simulink model "scheme1"  (R2024a)
settings: Solver=VariableStepAuto  StartTime=0.0  StopTime=inf  RelTol=1e-9
undefined symbols (not defined in the file): J, ke, km, R
libraries: instrumentseriallib x2
settings Model: Creator=alexivanov  LastModifiedBy=alexivanov

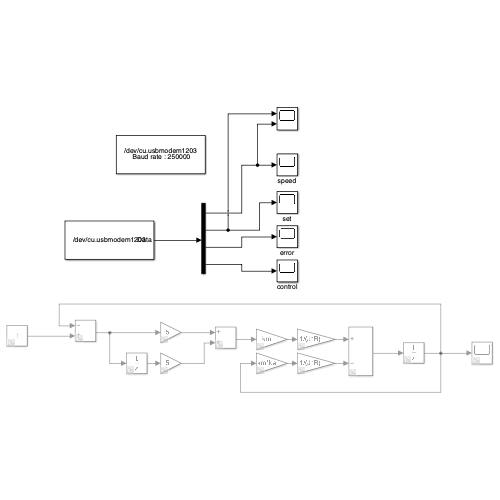
[thumbnail: Simulink's stored preview of the top-level diagram]
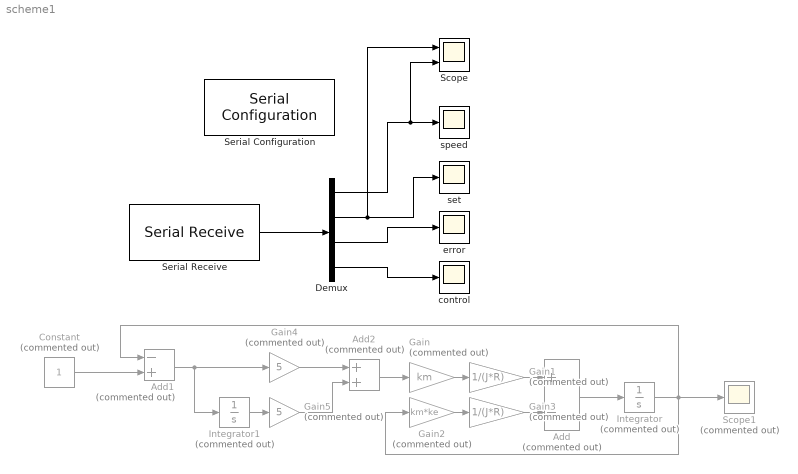
== system scheme1 ==
  Add : Sum  Commented=on  Inputs=+-
  Add1 : Sum  Commented=on  Inputs=-+
  Add2 : Sum  Commented=on
  Constant : Constant  Commented=on
  Demux : Demux
  Gain : Gain  Commented=on  Gain=km
  Gain1 : Gain  Commented=on  Gain=1/(J*R)
  Gain2 : Gain  Commented=on  Gain=km*ke
  Gain3 : Gain  Commented=on  Gain=1/(J*R)
  Gain4 : Gain  Commented=on  Gain=5
  Gain5 : Gain  Commented=on  Gain=5
  Integrator : Integrator  Commented=on
  Integrator1 : Integrator  Commented=on
  Scope : Scope  NumInputPorts=2
  Scope1 : Scope  Commented=on
  Serial Configuration : instrumentseriallib/Serial Configuration  Priority=-200000  PortSel=/dev/cu.usbmodem1203  Port=/dev/cu.usbmodem1203  ComPort=/dev/cu.usbmodem1203  BaudRate=250000  DataBits=8  Parity=none  StopBits=1  ByteOrder=little-endian  FlowControl=none  Timeout=10  SimulateUsing=Interpreted execution  BlockInModel=on  aMode=1
  Serial Receive : instrumentseriallib/Serial Receive  Priority=1  PortSel=/dev/cu.usbmodem1203  Port=/dev/cu.usbmodem1203  ComPort=/dev/cu.usbmodem1203  DataType=int16  SaveDataType=uint8  ToggleHeader=on  Header=[170 170]  ToggleDataSize=on  DataSize=[4 1]  ToggleTerminator=on  Terminator=Custom terminator  CustomTerminator=[255 255]  InputFormat=Column major  EnableBlockingMode=on  ActionDataUnavailable=Output last received value  ActionWhenDataUnavailable=Output last received value  CustomValue=0  SampleTime=0.01  SimulateUsing=Interpreted execution  BlockInModel=on  aMode=1
  control : Scope
  error : Scope
  set : Scope
  speed : Scope
  wires:
  Gain/1 -> Gain1/1
  Gain1/1 -> Add/1
  Gain2/1 -> Gain3/1
  Gain3/1 -> Add/2
  Add/1 -> Integrator/1
  Integrator/1 -> Add1/1, Scope1/1, Gain2/1
  Add1/1 -> Integrator1/1, Gain4/1
  Constant/1 -> Add1/2
  Integrator1/1 -> Gain5/1
  Add2/1 -> Gain/1
  Gain5/1 -> Add2/2
  Gain4/1 -> Add2/1
  Serial Receive/1 -> Demux/1
  Demux/1 -> Scope/2, speed/1
  Demux/2 -> Scope/1, set/1
  Demux/3 -> error/1
  Demux/4 -> control/1
